simulink model "digital_scale_with_control1"  (R2024b)
settings: Solver=VariableStepAuto  StartTime=0.0  StopTime=10.0  RelTol=1e-3
values from neighbouring files (symbols this model uses):
  c = 1500    [parameters.m]
  d = 8.5    [parameters.m]
  g = 9.81    [parameters.m]
  K_D = 20    [parameters.m]
  K_I = 8000    [parameters.m]
  K_P = 400    [parameters.m]
  KG = 5    [parameters.m]
  L = 20    [parameters.m]
  m = 0.02    [parameters.m]
  mp = 0.03    [parameters.m]
  R = 1    [parameters.m]
  umax = 15    [parameters.m]
  v0 = 0    [parameters.m]
  x0 = 0    [parameters.m]
settings Model: Creator=kavin  LastModifiedBy=kavin

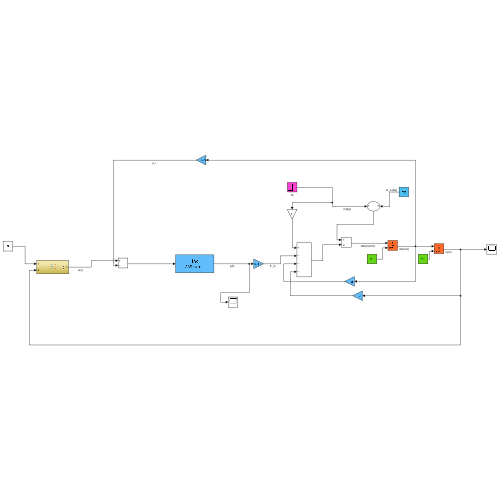
[thumbnail: Simulink's stored preview of the top-level diagram]
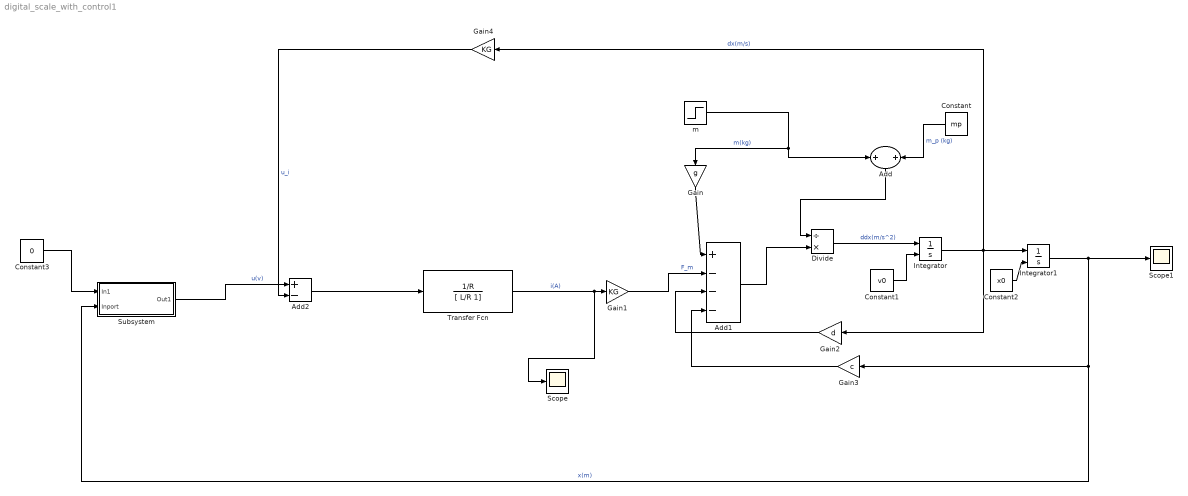
== system digital_scale_with_control1 ==
  Add : Sum
  Add1 : Sum  Inputs=+---
  Add2 : Sum  Inputs=+-
  Constant : Constant  Value=mp
  Constant1 : Constant  Value=v0
  Constant2 : Constant  Value=x0
  Constant3 : Constant  Value=0
  Divide : Product  Inputs=/*
  Gain : Gain  Gain=g
  Gain1 : Gain  Gain=KG
  Gain2 : Gain  Gain=d
  Gain3 : Gain  Gain=c
  Gain4 : Gain  Gain=KG
  Integrator : Integrator  InitialConditionSource=external
  Integrator1 : Integrator  InitialConditionSource=external
  Scope : Scope
  Scope1 : Scope
  Subsystem : Subsystem
  Transfer Fcn : TransferFcn  Numerator=1/R  Denominator=[ L/R 1]
  m : Step  After=m  SampleTime=0
  wires:
  Constant1/1 -> Integrator/2
  Add/1 -> Divide/1
  m/1 -> Gain/1, Add/1  "m(kg)"
  Gain4/1 -> Add2/2  "u_i"
  Gain3/1 -> Add1/4
  Constant/1 -> Add/2  "m_p (kg)"
  Gain/1 -> Add1/1
  Transfer Fcn/1 -> Scope/1, Gain1/1  "i(A)"
  Integrator1/1 -> Subsystem/2(Inport), Gain3/1, Scope1/1  "x(m)"
  Gain1/1 -> Add1/2  "F_m"
  Divide/1 -> Integrator/1  "ddx(m/s^2)"
  Gain2/1 -> Add1/3
  Integrator/1 -> Gain4/1, Gain2/1, Integrator1/1  "dx(m/s)"
  Constant2/1 -> Integrator1/2
  Add1/1 -> Divide/2
  Subsystem/1(Out1) -> Add2/1  "u(v)"
  Constant3/1 -> Subsystem/1(In1)
  Add2/1 -> Transfer Fcn/1

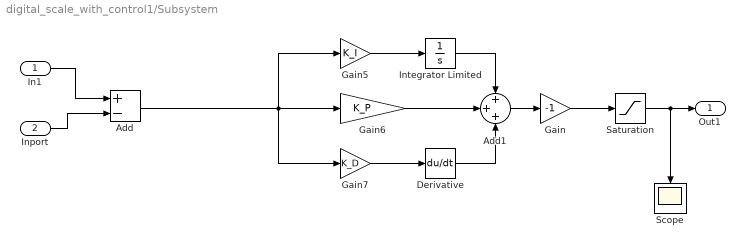
== system digital_scale_with_control1/Subsystem ==
  In1 : Inport
  Inport : Inport  Port=2
  Add : Sum  Inputs=+-
  Add1 : Sum  Inputs=+++
  Derivative : Derivative
  Gain : Gain  Gain=-1
  Gain5 : Gain  Gain=K_I
  Gain6 : Gain  Gain=K_P
  Gain7 : Gain  Gain=K_D
  Integrator Limited : Integrator  LimitOutput=on  UpperSaturationLimit=umax  LowerSaturationLimit=-umax
  Saturation : Saturate  UpperLimit=umax  LowerLimit=-umax
  Scope : Scope
  Out1 : Outport
  wires:
  In1/1 -> Add/1
  Inport/1 -> Add/2
  Gain7/1 -> Derivative/1
  Saturation/1 -> Out1/1, Scope/1
  Gain6/1 -> Add1/2
  Add1/1 -> Gain/1
  Gain5/1 -> Integrator Limited/1
  Integrator Limited/1 -> Add1/1
  Gain/1 -> Saturation/1
  Add/1 -> Gain5/1, Gain7/1, Gain6/1
  Derivative/1 -> Add1/3
